simulink model "lead_rapid_increase_space"  (R2025a)
settings: Solver=VariableStepAuto  StartTime=0.0  StopTime=10.0  RelTol=1e-3
settings Model: Creator=sanborkl  LastModifiedBy=sanborkl

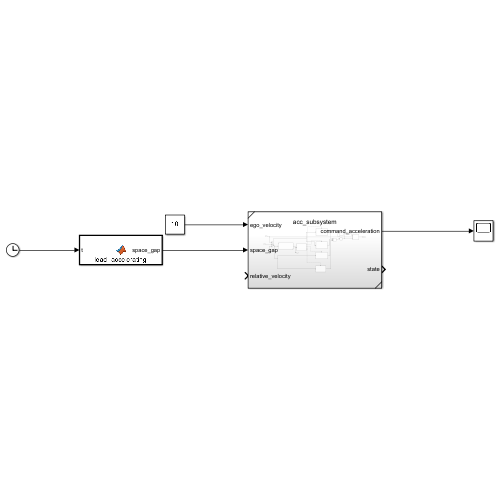
[thumbnail: Simulink's stored preview of the top-level diagram]
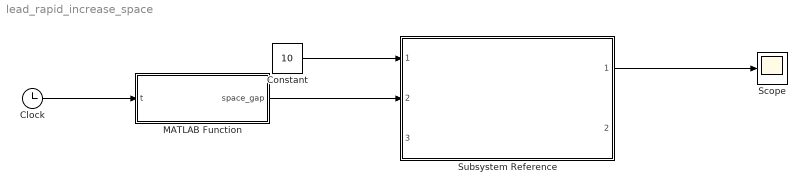
== system lead_rapid_increase_space ==
  Clock : Clock
  Constant : Constant  Value=10
  MATLAB Function : MATLAB Function  TreatAsAtomicUnit=on
  Scope : Scope
      settings: ActiveDisplayYMinimum=-0.18749999999999994  ActiveDisplayYMaximum=1.6875
  Subsystem Reference : Subsystem  ReferencedSubsystem=acc_subsystem
  wires:
  Constant/1 -> Subsystem Reference/1
  MATLAB Function/1(space_gap) -> Subsystem Reference/2
  Clock/1 -> MATLAB Function/1(t)
  Subsystem Reference/1 -> Scope/1

== matlab function lead_rapid_increase_space/MATLAB Function ==
  data: t input; space_gap output
function space_gap = lead_accelerating(t)

space_gap = 20 + 5 * t;
